simulink model "TrainingModel"  (R2024a)
settings: Solver=VariableStepAuto  StartTime=0.0  StopTime=1  RelTol=1e-3
libraries: dspsrcs4 x1
settings Model: Creator=pvenupra  LastModifiedBy=pvenupra

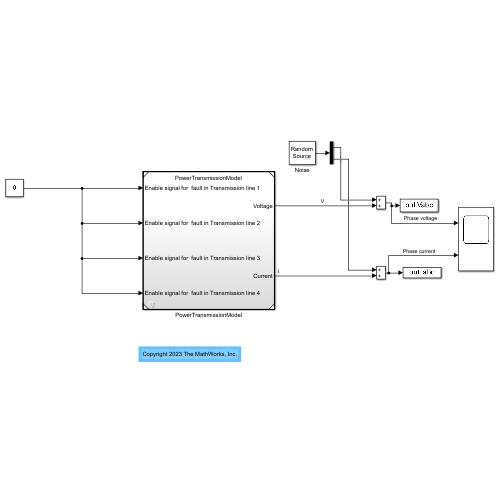
[thumbnail: Simulink's stored preview of the top-level diagram]
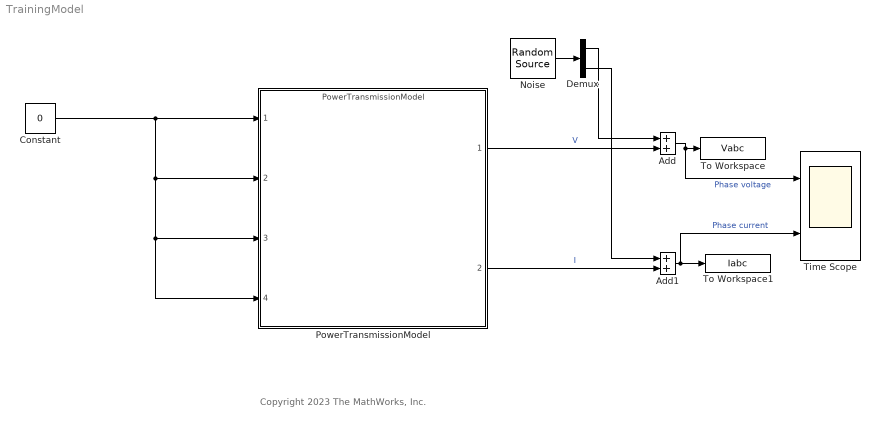
== system TrainingModel ==
  note: Copyright 2023 The MathWorks, Inc.
  Add : Sum
  Add1 : Sum
  Constant : Constant  Value=0  SampleTime=0.025
  Demux : Demux  Outputs=2
  Noise : dspsrcs4/Random Source  SrcType=Gaussian  MinVal=0  MaxVal=1  MeanVal=0  VarVal=[1000 .01]  RepMode=Specify seed  rawSeed=1  IsInherit=off  SampFrame=1  DataType=double  OutComplex=Real  SampTime=1e-4  SimulateUsing=Interpreted execution
  PowerTransmissionModel : ModelReference  ModelNameDialog=PowerTransmissionModel.slx  SimulationMode=Normal  ModelReferenceVersion=1.70
  Time Scope : Scope  NumInputPorts=2
  To Workspace : ToWorkspace  VariableName=Vabc  SampleTime=-1
      settings: Save2DSignal=2-D array (concatenate along first dimension)
  To Workspace1 : ToWorkspace  VariableName=Iabc  SampleTime=-1
      settings: Save2DSignal=2-D array (concatenate along first dimension)
  wires:
  Constant/1 -> PowerTransmissionModel/3, PowerTransmissionModel/4, PowerTransmissionModel/2, PowerTransmissionModel/1
  Demux/2 -> Add1/1
  PowerTransmissionModel/2 -> Add1/2  "I"
  PowerTransmissionModel/1 -> Add/2  "V"
  Noise/1 -> Demux/1
  Add1/1 -> Time Scope/2, To Workspace1/1  "Phase current"
  Demux/1 -> Add/1
  Add/1 -> Time Scope/1, To Workspace/1  "Phase voltage"
